simulink model "computeTau"  (Simulink 7.9)
settings: Solver=FixedStepDiscrete  StartTime=0.0  StopTime=5  FixedStep=0.01  RelTol=1e-3
PreLoadFcn:
  | robotName = 'icubGazeboSim';
  | localName = 'SimulinkiCubGazeboSim';
InitFcn:
  | robotName = 'icubGazeboSim';
  | localName = 'SimulinkiCubGazeboSim';
libraries: WBCLibrary x10, simulink x1, dspsigops x1
settings Model: Creator=iron  LastModifiedBy=jorhabib
settings DebuggingCC: FcnCallInpInsideContextMsg=Use local settings
settings CodeAppCC: CustomSymbolStrType=$N$R$M_T
settings GRTTargetCC: CodeReplacementLibrary=C89/C90 (ANSI)  CombineOutputUpdateFcns=off  GRTInterface=on

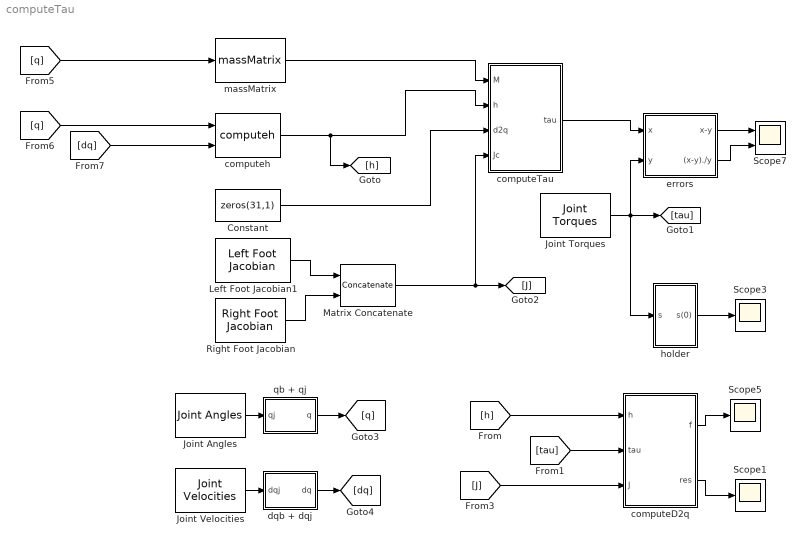
== system computeTau ==
  Constant : Constant  Value=zeros(31,1)
  Joint Angles : WBCLibrary/wholeBodyStates/Joint Angles  robotName=robotName  localName=localName
  Joint Torques : WBCLibrary/wholeBodyStates/Joint Torques  robotName=robotName  localName=localName
  Joint Velocities : WBCLibrary/wholeBodyStates/Joint Velocities  robotName=robotName  localName=localName
  Left Foot Jacobian1 : WBCLibrary/wholeBodyModel/Jacobians/Left Foot Jacobian  robotName=robotName  localName=localName
  Matrix Concatenate : Concatenate  Mode=Multidimensional array
  Right Foot Jacobian : WBCLibrary/wholeBodyModel/Jacobians/Right Foot Jacobian  robotName=robotName  localName=localName
  Scope1 : Scope
      settings: YMin=-1.5  YMax=5.5
  Scope3 : Scope
      settings: YMin=-5.5  YMax=3  SaveName=ScopeData3
  Scope5 : Scope
      settings: YMin=-10  YMax=120
  Scope7 : Scope  NumInputPorts=2
      settings: YMin=-0.45~-5  YMax=0.55~5  SaveName=ScopeData7
  computeD2q : MATLAB Function  TreatAsAtomicUnit=on
      settings: PermitHierarchicalResolution=ParametersOnly
  computeTau : MATLAB Function  TreatAsAtomicUnit=on
      settings: PermitHierarchicalResolution=ParametersOnly
  computeh : WBCLibrary/wholeBodyModel/Dynamics/computeh  val=7  robotname=robotName  localname=localName
  dqb + dqj : Subsystem
  errors : Subsystem
  holder : Subsystem
  massMatrix : WBCLibrary/wholeBodyModel/Dynamics/massMatrix  val=8  robotname=robotName  localname=localName
  qb + qj : Subsystem
  wires:
  massMatrix/1 -> computeTau/1(M)
  computeh/1 -> [h], computeTau/2(h)
  Joint Torques/1 -> errors/2(y), holder/1(s), [tau]
  holder/1(s(0)) -> Scope3/1
  computeTau/1(tau) -> errors/1(x)
  Constant/1 -> computeTau/3(d2q)
  errors/1(x-y) -> Scope7/1
  Matrix Concatenate/1 -> computeTau/4(Jc), [J]
  Right Foot Jacobian/1 -> Matrix Concatenate/2
  Left Foot Jacobian1/1 -> Matrix Concatenate/1
  [tau] -> computeD2q/2(tau)
  computeD2q/2(res) -> Scope1/1
  computeD2q/1(f) -> Scope5/1
  [h] -> computeD2q/1(h)
  [J] -> computeD2q/3(J)
  Joint Angles/1 -> qb + qj/1(qj)
  Joint Velocities/1 -> dqb + dqj/1(dqj)
  qb + qj/1(q) -> [q]
  dqb + dqj/1(dq) -> [dq]
  [q] -> massMatrix/1
  [q] -> computeh/1
  [dq] -> computeh/2
  errors/2((x-y)./y) -> Scope7/2

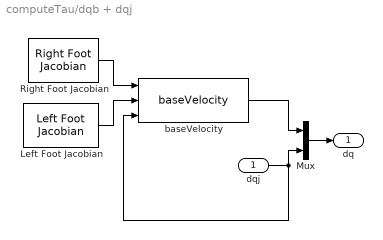
== system computeTau/dqb + dqj ==
  dqj : Inport
  Left Foot Jacobian : WBCLibrary/wholeBodyModel/Jacobians/Left Foot Jacobian  robotName=robotName  localName=localName
  Mux : Mux  Inputs=2
  Right Foot Jacobian : WBCLibrary/wholeBodyModel/Jacobians/Right Foot Jacobian  robotName=robotName  localName=localName
  baseVelocity : WBCLibrary/Utilities/baseVelocity
  dq : Outport
  wires:
  Left Foot Jacobian/1 -> baseVelocity/2
  Right Foot Jacobian/1 -> baseVelocity/1
  baseVelocity/1 -> Mux/1
  dqj/1 -> baseVelocity/3, Mux/2
  Mux/1 -> dq/1

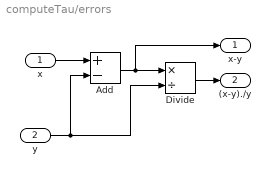
== system computeTau/errors ==
  x : Inport
  y : Inport  Port=2
  Add : Sum  Inputs=+-
  Divide : Product  Inputs=*/
  x-y : Outport
  (x-y)./y : Outport  Port=2
  wires:
  Add/1 -> x-y/1, Divide/1
  x/1 -> Add/1
  y/1 -> Add/2, Divide/2
  Divide/1 -> (x-y)./y/1

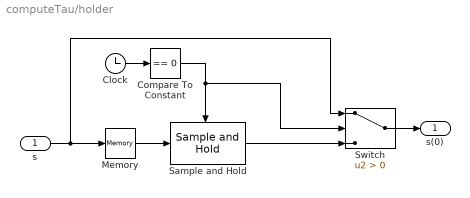
== system computeTau/holder ==
  s : Inport
  Clock : Clock
  Compare To Constant : simulink/Logic and Bit Operations/Compare To Constant  relop===  const=0  OutDataTypeStr=boolean
  Memory : Memory
  Sample and Hold : dspsigops/Sample and Hold  trig=Falling edge  initCond=0  latchinput=off
  Switch : Switch  Criteria=u2 > Threshold
  s(0) : Outport
  wires:
  s/1 -> Switch/1, Memory/1
  Clock/1 -> Compare To Constant/1
  Compare To Constant/1 -> Sample and Hold/Trigger, Switch/2
  Sample and Hold/1 -> Switch/3
  Switch/1 -> s(0)/1
  Memory/1 -> Sample and Hold/1

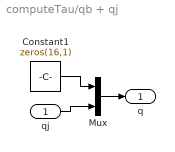
== system computeTau/qb + qj ==
  qj : Inport
  Constant1 : Constant  Value=zeros(16,1)
  Mux : Mux  Inputs=2
  q : Outport
  wires:
  Mux/1 -> q/1
  Constant1/1 -> Mux/1
  qj/1 -> Mux/2

== matlab function computeD2q ==
  data: h input double; tau input double; J input double; f output double; res output double
function [f, res] = fcn(h, tau, J)

% Francesco Nori
% Genova 10 Marzo 2014
% CODYCO project
%
% This code computes the d2q given the currently applied torques,
% assuming contacts at both feet.
%
% M d2q + h - J' f = S' tau  
%
% with the constraints being described as:
%
% J dq = 0
%
% J d2q + dJdq= 0

[~, n] = size(J);
S = [zeros(n-6, 6), eye(n-6)];
f = -pinv(J')*(S'*tau - h);
res = J'*f + S'*tau - h;

% res = h(7:31) - tau;
% f = 0;

== matlab function computeTau ==
  data: M input double; h input double; d2q input double; tau output double; Jc input double
function tau  = fcn(M, h, d2q, Jc)

% Francesco Nori
% Genova 6 Marzo 2014
% CODYCO project
%
% This code computes the torques tau necessary to obtain a desired
% acceleration d2q in a kinematic chain with contacts. These 
% computations are described in (DelPrete,2013) Ph.D. thesis
% and can be found also in [Aghili 2005; Righetti et al. 2011]. It can
% be shown that:
%
% tau = pinv(Nc' S') Nc (M d2q  + h)  
%
% with Nc = (I-pinv(Jc)Jc) and the constraints being described as:
%
% Jc dq = 0
%
% Jc d2q + dJcdq= 0

[~, n] = size(Jc);
n = n - 6;
S = [zeros(n,6) eye(n)];

Nc = (eye(n+6)-pinv(Jc, 1e-2)*Jc);
tau = pinv(Nc' * S', 1e-2) * Nc *(M * d2q  + h);
